simulink model "qaff2"  (Simulink 3.00)
settings: Solver=ode45  SolverMode=SingleTasking  StartTime=0.0  StopTime=40  MaxStep=0.010  RelTol=1e-3  AbsTol=1e-3
settings Model: TimeSaveName=t  SaveOutput=off

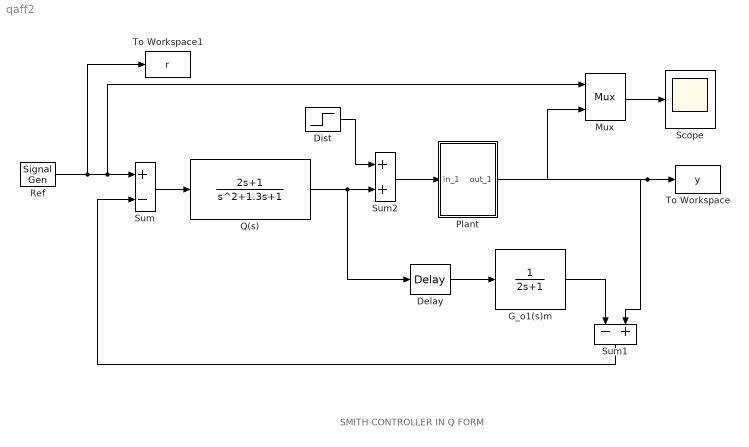
== system qaff2 ==
  note: SMITH CONTROLLER IN Q FORM
  Delay : TransportDelay  DelayTime=1  InitialInput=0  BufferSize=4096
  Dist : Step  Time=10  Before=0  After=1  SampleTime=0
  G_o1(s)m : TransferFcn  Numerator=[1]  Denominator=[2 1]
  Mux : Mux  Inputs=2
      settings: DisplayOption=none
  Plant : Subsystem
      mask Type: Plant
      mask Display: disp('Plant')
  Q(s) : TransferFcn  Numerator="[ 2  1]"  Denominator=[1 1.3 1]
  Ref : SignalGenerator  WaveForm=square  Amplitude=1.000000  Frequency=0.150000  Units=rad/sec
  Scope : Scope
      settings: TickLabels=on  TimeRange=40.000000  YMin=-2  YMax=2  SaveToWorkspace=off  SaveName=ScopeData  DataFormat=Matrix
  Sum : Sum  Inputs=+-  SaturateOnIntegerOverflow=on
  Sum1 : Sum  Orientation=down  Inputs=-+  SaturateOnIntegerOverflow=on
  Sum2 : Sum  Inputs=++  SaturateOnIntegerOverflow=on
  To Workspace : ToWorkspace  VariableName=y  SampleTime=0  SaveFormat=Matrix
      settings: Buffer=10000
  To Workspace1 : ToWorkspace  VariableName=r  SampleTime=0  SaveFormat=Matrix
      settings: Buffer=10000
  wires:
  Sum2/1 -> Plant/1(in_1)
  Dist/1 -> Sum2/1
  Sum/1 -> Q(s)/1
  Delay/1 -> G_o1(s)m/1
  Mux/1 -> Scope/1
  G_o1(s)m/1 -> Sum1/1
  Sum1/1 -> Sum/2
  Ref/1 -> To Workspace1/1, Sum/1, Mux/1
  Plant/1(out_1) -> To Workspace/1, Sum1/2, Mux/2
  Q(s)/1 -> Sum2/2, Delay/1

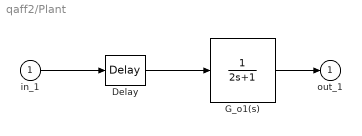
== system qaff2/Plant ==
  in_1 : Inport  Port=1  PortWidth=-1  SampleTime=-1  DataType=auto
      settings: SignalType=auto
  Delay : TransportDelay  DelayTime=1  InitialInput=0  BufferSize=4096
  G_o1(s) : TransferFcn  Numerator=[1]  Denominator=[2 1]
  out_1 : Outport  Port=1  InitialOutput=0
  wires:
  Delay/1 -> G_o1(s)/1
  in_1/1 -> Delay/1
  G_o1(s)/1 -> out_1/1
